simulink subsystem "DC_motor_and_gearbox"  (R2024b)
settings: Solver=VariableStepAuto  StartTime=0.0  StopTime=10.0  RelTol=1e-3
undefined symbols (not defined in the file or in its folder): Bl, Bm, Jl, Jm, ke, Kt, L, N, rads2rpm, Req, tausf
settings Model: Creator=Federico Bergami  LastModifiedBy=Riccardo Grosso

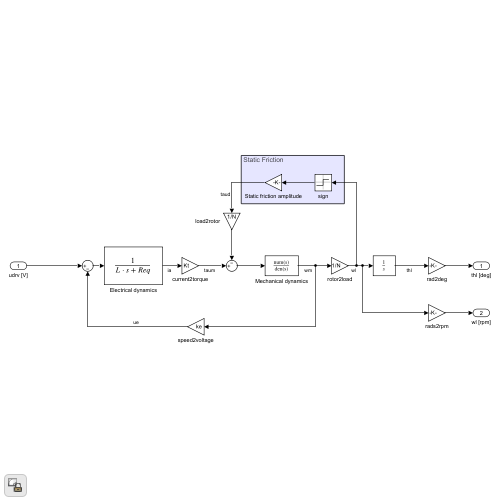
[thumbnail: Simulink's stored preview of the top-level diagram]
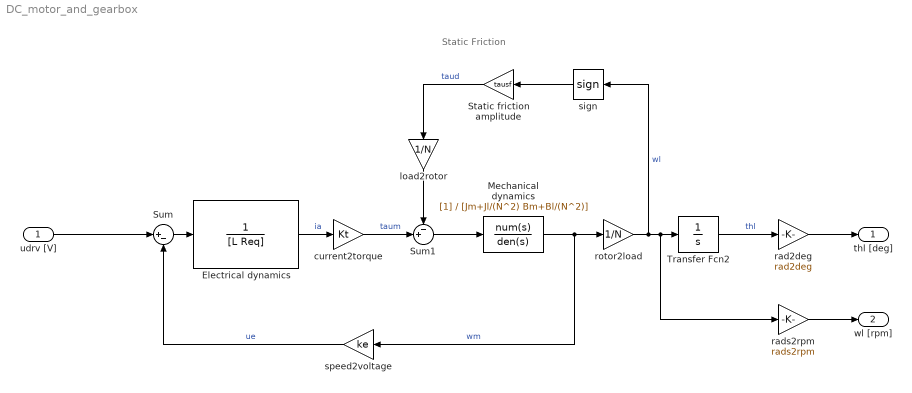
== system DC_motor_and_gearbox ==
  note: Static Friction
  udrv [V] : Inport
  Electrical dynamics : TransferFcn  Denominator=[L Req]
  Mechanical dynamics : TransferFcn  Denominator=[Jm+Jl/(N^2) Bm+Bl/(N^2)]
  Static friction amplitude : Gain  Gain=tausf
  Sum : Sum  Inputs=|+-
  Sum1 : Sum  Inputs=-+|
  Transfer Fcn2 : TransferFcn  Denominator=[1 0]
  current2torque : Gain  Gain=Kt
  load2rotor : Gain  Gain=1/N
  rad2deg : Gain  Gain=rad2deg
  rads2rpm : Gain  Gain=rads2rpm
  rotor2load : Gain  Gain=1/N
  sign : Signum  ZeroCross=off
  speed2voltage : Gain  Gain=ke
  thl [deg] : Outport
  wl [rpm] : Outport  Port=2
  wires:
  rad2deg/1 -> thl [deg]/1
  rads2rpm/1 -> wl [rpm]/1
  load2rotor/1 -> Sum1/1
  Sum1/1 -> Mechanical dynamics/1
  sign/1 -> Static friction amplitude/1
  rotor2load/1 -> sign/1, rads2rpm/1, Transfer Fcn2/1  "wl"
  speed2voltage/1 -> Sum/2  "ue"
  Static friction amplitude/1 -> load2rotor/1  "taud"
  udrv [V]/1 -> Sum/1
  Mechanical dynamics/1 -> speed2voltage/1, rotor2load/1  "wm"
  current2torque/1 -> Sum1/2  "taum"
  Electrical dynamics/1 -> current2torque/1  "ia"
  Sum/1 -> Electrical dynamics/1
  Transfer Fcn2/1 -> rad2deg/1  "thl"
